simulink model "a"  (R2022a)
settings: Solver=VariableStepAuto  StartTime=0.0  StopTime=0.1  RelTol=1e-3
libraries: commrandsrc3 x1, dspsrcs4 x1
(part 1 of 4)
settings Model: Creator=Sepiamw  LastModifiedBy=asusiran
settings DebuggingCC: UnconnectedInputMsg=warning  UnconnectedOutputMsg=warning  UnconnectedLineMsg=warning
settings RTWCC: DLArmComputeVersion=19.05

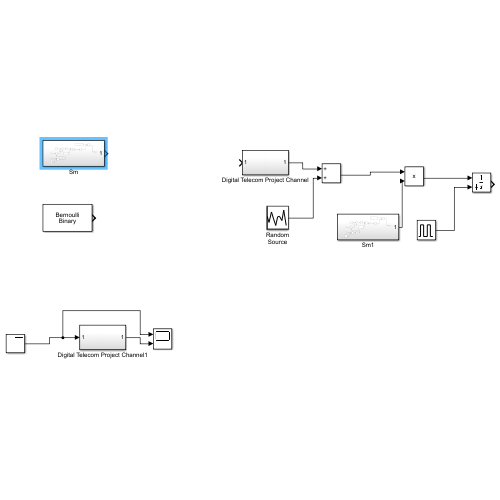
[thumbnail: Simulink's stored preview of the top-level diagram]
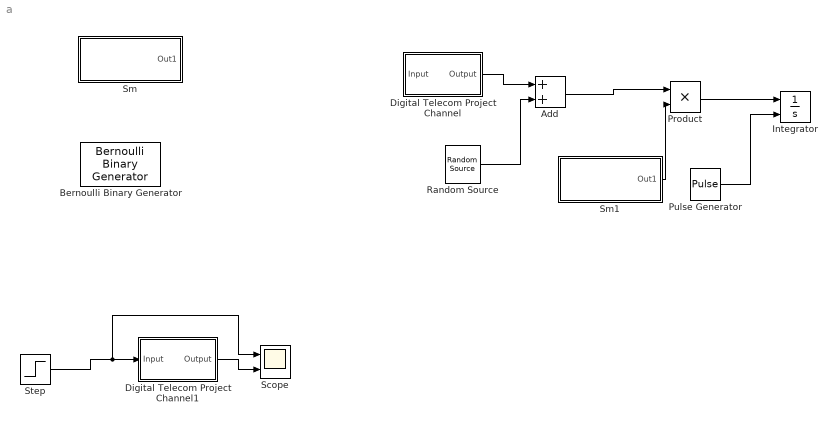
== system a ==
  Add : Sum
  Bernoulli Binary Generator : commrandsrc3/Bernoulli Binary Generator  ProbabilityOfZero=0.5  SeedSource=Auto  Seed=0  SampleTime=1  SamplesPerFrame=1  OutputDataType=double  SimulateUsing=Interpreted execution
  Digital Telecom Project Channel : Subsystem  Tag=FilterWizardSubSystem
      settings: ErrorFcn=dspFilterRealizedInBasicElemsAlgLoopErrFcnCallback
  Digital Telecom Project Channel1 : Subsystem  Tag=FilterWizardSubSystem
      settings: ErrorFcn=dspFilterRealizedInBasicElemsAlgLoopErrFcnCallback
  Integrator : Integrator  ExternalReset=rising
  Product : Product
  Pulse Generator : DiscretePulseGenerator  PulseType=Time based  Period=1e-3  PulseWidth=5
  Random Source : dspsrcs4/Random Source  SrcType=Uniform  NormMethod=Ziggurat  CltLength=12  MinVal=0  MaxVal=100  MeanVal=0  VarVal=1  RepMode=Not repeatable  rawSeed=1  IsInherit=off  SampMode=Discrete  SampTime=1e-5  SampFrame=1  DataType=Double  OutComplex=Real  OutputFrames=off
  Scope : Scope  NumInputPorts=2
  Sm : Subsystem
  Sm1 : Subsystem
  Step : Step  Time=0  SampleTime=0
  wires:
  Digital Telecom Project Channel/1(Output) -> Add/1
  Random Source/1 -> Add/2
  Add/1 -> Product/1
  Sm1/1(Out1) -> Product/2
  Product/1 -> Integrator/1
  Pulse Generator/1 -> Integrator/2
  Step/1 -> Scope/1, Digital Telecom Project Channel1/1(Input)
  Digital Telecom Project Channel1/1(Output) -> Scope/2
